simulink model "CubeX_Fast_MPC_2D"  (R2016b)
settings: Solver=FixedStepDiscrete  StartTime=0.0  StopTime=inf  FixedStep=Ts.base  RelTol=1e-3
PreLoadFcn:
  | waijung.modelPreload; % Required for working with Waijung Blockset. Do not remove.
InitFcn:
  | cubeparameters
undefined symbols (not defined in the file or in its folder): CPHA_1Edge, CPOL_Low, deg_, Duplex, FirstBit_MSB, Full, g, imu, Link, LQFP100, ST, STM32F407VG, STM32F4DISCOVERY, Ts
libraries: simulink x47, stm32f4_i2c_lib x12, stm32f4_io_lib x5, stm32f4_spi_lib x4, cube_lib x3, BC_USB x2, stm32f4_adc_lib x1, stm32f4_device_config_lib x1
(part 1 of 3)
CloseFcn:
  | waijung.modelClose; % Required for working with Waijung Blockset. Do not remove.
settings Model: Creator=Hi  LastModifiedBy=Wall
settings DataIOCC: LimitDataPoints=on  SaveFormat=Array
settings OptimizationCC: LifeSpan=1
settings DebuggingCC: AllowSymbolicDim=off  SFUnexpectedBacktrackingDiag=warning  SFNoUnconditionalDefaultTransitionDiag=warning  SFExecutionAtInitializationDiag=none
settings HardwareCC: ProdBitPerPointer=32  ProdBitPerSizeT=32  ProdBitPerPtrDiffT=32  ProdLargestAtomicFloat=None  ProdIntDivRoundTo=Undefined  ProdWordSize=32  ProdHWDeviceType=ARM Compatible->Cortex - M4  TargetEndianess=LittleEndian  TargetHWDeviceType=ARM Compatible->Cortex - M4
settings ModelReferenceCC: PropagateSignalLabelsOutOfModel=off
settings RTWCC: SystemTargetFile=stm32f4.tlc  GenerateMakefile=off  TemplateMakefile=ert_default_tmf  Description=STM32F4 Target
settings CodeAppCC: ForceParamTrailComments=on  IgnoreCustomStorageClasses=off  OperatorAnnotations=on  SimulinkDataObjDesc=on  InsertBlockDesc=on  MATLABSourceComments=on
settings STFCustomTargetCC: ModelReferenceCompliant=off  CombineOutputUpdateFcns=on  ERTCustomFileBanners=on  SupportContinuousTime=off  SupportNonInlinedSFcns=off  RemoveResetFunc=on  MATLABClassNameForMDSCustomization=Simulink.SoftwareTarget.ERTCustomization  GRTInterface=off  SystemTargetFile=stm32f4.tlc
settings ERTTargetCC: ModelReferenceCompliant=off  ParMdlRefBuildCompliant=off  CompOptLevelCompliant=off  ConcurrentExecutionCompliant=off  ERTFirstTimeCompliant=off  ModelStepFunctionPrototypeControlCompliant=off  CPPClassGenCompliant=off  UseToolchainInfoCompliant=off  ERTSrcFileBannerTemplate=stm32f4_code_template.cgt  ERTHdrFileBannerTemplate=stm32f4_code_template.cgt  ERTDataSrcFileTemplate=stm32f4_code_template.cgt  ERTDataHdrFileTemplate=stm32f4_code_template.cgt  ERTCustomFileTemplate=stm32f4_file_process.tlc  ConvertIfToSwitch=off  SuppressUnreachableDefaultCases=off
settings ConfigComp: CovMetricSettings=dw  CovHtmlReporting=on  CovSaveCumulativeToWorkspaceVar=on  CovSaveSingleToWorkspaceVar=on  CovExternalEMLEnable=off

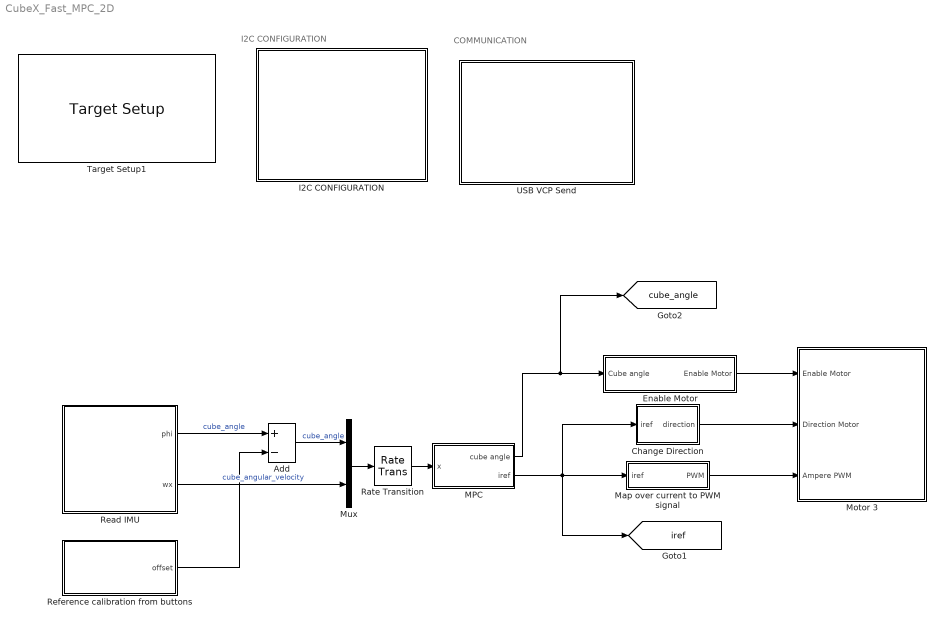
== system CubeX_Fast_MPC_2D ==
  note: COMMUNICATION
  note: I2C CONFIGURATION
  Add : Sum  Inputs=+-
  Change Direction : Subsystem
  Enable Motor : Subsystem  SystemSampleTime=Ts.controller
  I2C CONFIGURATION : Subsystem
  MPC : Subsystem  SystemSampleTime=Ts.controller
      settings: MinAlgLoopOccurrences=on
  Map over current to PWM signal : Subsystem
  Motor 3 : Subsystem
  Mux : Mux  Inputs=2
  Rate Transition : RateTransition  OutPortSampleTime=Ts.controller
  Read IMU : Subsystem
  Reference calibration from buttons : Subsystem
  Target Setup1 : stm32f4_device_config_lib/Target Setup  Priority=100  compiler=GNU ARM  previous_compiler=GNU ARM  mcu=STM32F407VG (LQFP100); STM32F4DISCOVERY  mcustr=STM32F407VG  clockconfig=STM32F4DISCOVERY Default (HSEOSC-8MHz/HCLK-168MHz)  system_stm32f4xx_c_path=C:\waijung15_04a\targets\stm32f4_target\stm32f4\utils\STM32F4xx_AN3988_V1.0.1\stm32f4_default\hseosc8mhz  showmemoryconfiguration=off  stacksize=0x400  heapsize=0x200  enableautocompiledownload=on  fullchiperase=off  programmerinterface=ST-Link  editctrlstr=on  compilercontrolstr=$(patsubst %, -I%, .) -mcpu=cortex-m4 -mthumb -mthumb-interwork -mfloat-abi=hard -mfpu=fpv4-sp-d16 -ffast-math -Wall -Wextra -Ofast  assemblercontrolstr=$(patsubst %, -I%, .) -mcpu=cortex-m4 -mthumb -mthumb-interwork -mfloat-abi=hard -mfpu=fpv4-sp-d16 -ffast-math -Wall -Wextra -Ofast -Wa,-amhls=$(<:.s=.lst) -D__STACK_SIZE=$(STACK_SIZE) -D__HEAP_SIZE=$(HEAP_SIZE)  linkercontrolstr=-T$(LD_SCRIPT) -g -Wl,-Map=$(MAP),--cref,--no-warn-mismatch -mcpu=cortex-m4 -mthumb -mthumb-interwork -mfloat-abi=hard -mfpu=fpv4-sp-d16  runafterdownload=on  execprofile=None  profileruart=1  profilerbaud=115200  profilertxpin=Not used  profilerinitstr=0.002,168000000,336000,115200,0  manualsetsampletime=on  sampletime=0.002  blockid=TargetSetup1  systickreloadvalue=336000  hseval=8000000  lastprofileruart=1  hclk=168000000  flashorigin=0x8000000  flashlength=1M  ramorigin=0x20000000  ramlength=112k  useextram=off
  USB VCP Send : Subsystem
  tag scope: cube_angle=global, iref=global
  wires:
  Read IMU/2(wx) -> Mux/2  "cube_angular_velocity"
  Reference calibration from buttons/1(offset) -> Add/2
  Add/1 -> Mux/1  "cube_angle"
  Read IMU/1(phi) -> Add/1  "cube_angle"
  MPC/2(iref) -> [iref], Change Direction/1(iref), Map over current to PWM signal/1(iref)
  Map over current to PWM signal/1(PWM) -> Motor 3/3(Ampere PWM)
  Change Direction/1(direction) -> Motor 3/2("Direction Motor ")
  Enable Motor/1(Enable Motor) -> Motor 3/1(Enable Motor)
  Mux/1 -> Rate Transition/1
  Rate Transition/1 -> MPC/1(x)
  MPC/1(cube angle) -> [cube_angle], Enable Motor/1(Cube angle)

== system CubeX_Fast_MPC_2D/Change Direction ==
  iref : Inport
  Compare To Zero : simulink/Logic and Bit Operations/Compare To Zero  relop=<=  OutDataTypeStr=boolean
  Logical Operator : Logic  Operator=NOT  AllPortsSameDT=off  OutDataTypeStr=boolean
  direction : Outport
  wires:
  Compare To Zero/1 -> Logical Operator/1
  iref/1 -> Compare To Zero/1
  Logical Operator/1 -> direction/1

== system CubeX_Fast_MPC_2D/Enable Motor ==
  note: When the angle is abs of 6 degrees, Motor is enabled
  Cube angle : Inport
  Abs1 : Abs
  Compare To Constant : simulink/Logic and Bit Operations/Compare To Constant  relop=<=  const=deg2rad(3)  OutDataTypeStr=boolean
  Enable Motor : Outport
  wires:
  Abs1/1 -> Compare To Constant/1
  Cube angle/1 -> Abs1/1
  Compare To Constant/1 -> Enable Motor/1

== system CubeX_Fast_MPC_2D/I2C CONFIGURATION ==
  I2C Master Setup1 : S-Function  FunctionName=stm32f4_i2c  Parameters=configuration,module,transfer,clkspeed,timeout,sdapin,sclpin,writecount,readcount,inputtypearray,outputtypearray,confstr,sampletime,sampletimestr,blockid  SFunctionDeploymentMode=off  EnableBusSupport=off  mask(stm32f4_i2c){configuration=Setup, module=3, lastmodule=3, transfer=Blocking, dutycycle=TLow/THigh = 2, clkspeed=400, timeout=25, writecount=0, readcount=0, sdapin=C9, sclpin=A8, waitwritetime=0, inputtypearray=[0], outputtypearray=[0], confstr=["C","9","A","8","1","3","4","2","I2C_DutyCycle_2","0","off"], sampletime=-1, sampletimestr=0.002, blockid=I2CCONFIGURATIONI2CMasterSetup1}
      mask prompts: module "I2C Module"; lastmodule "Last module"; transfer "Transfer mode"; dutycycle "Duty cycle in fast mode"; clkspeed "Clock speed (kHz)"; timeout "Timeout (ms)"; writecount "Bytes write count"; readcount "Bytes read count"; sdapin "SDA pin"; sclpin "SCL pin"; waitwritetime "Wait write time (ms), default is 0"; inputtypearray "Input type array"; outputtypearray "Output type array"; confstr "Configuration string"; sampletime "Sample time (sec)"; sampletimestr "Compiled sample time (sec) in string"
      mask init:
      | stm32f4_i2c_callback('init');
      mask Help: web(fullfile(waijungdocroot,'stm32f4_i2c_setup.htm'), '-browser')
      mask TypeOptions configuration: Setup | Transaction
      mask Callback configuration: stm32f4_i2c_callback('configuration');
      mask TypeOptions module: 1 | 2 | 3
      mask Callback module: stm32f4_i2c_callback('module');
      mask TypeOptions transfer: Blocking | Non-blocking
      mask TypeOptions dutycycle: TLow/THigh = 16/9 | TLow/THigh = 2
      mask Callback dutycycle: stm32f4_i2c_callback('dutycycle');
      mask Callback writecount: stm32f4_i2c_callback('writecount');
      mask Callback readcount: stm32f4_i2c_callback('readcount');
      mask TypeOptions sdapin: - | C9
      mask Callback sdapin: stm32f4_i2c_callback('sdapin');
      mask TypeOptions sclpin: - | A8
      mask Callback sclpin: stm32f4_i2c_callback('sclpin');
      mask Callback confstr: stm32f4_i2c_callback('confstr');
      mask Callback sampletime: stm32f4_i2c_callback('sampletime');
      mask Callback sampletimestr: stm32f4_i2c_callback('sampletimestr');
      mask Callback blockid: stm32f4_i2c_callback('blockid');
      mask Display: text(0.5, 0.5, 'Module: I2C3\nClock: 400kHz\nSDA/SCL Pin: C9/A8','ver','middle','hor','center');
  I2C Master Setup2 : S-Function  FunctionName=stm32f4_i2c  Parameters=configuration,module,transfer,clkspeed,timeout,sdapin,sclpin,writecount,readcount,inputtypearray,outputtypearray,confstr,sampletime,sampletimestr,blockid  SFunctionDeploymentMode=off  EnableBusSupport=off  mask(stm32f4_i2c){configuration=Setup, module=1, lastmodule=1, transfer=Blocking, dutycycle=TLow/THigh = 2, clkspeed=400, timeout=25, writecount=0, readcount=0, sdapin=B9, sclpin=B6, waitwritetime=0, inputtypearray=[0], outputtypearray=[0], confstr=["B","9","B","6","1","1","6","0","I2C_DutyCycle_2","0","off"], sampletime=-1, sampletimestr=0.002, blockid=I2CCONFIGURATIONI2CMasterSetup2}
      mask prompts: module "I2C Module"; lastmodule "Last module"; transfer "Transfer mode"; dutycycle "Duty cycle in fast mode"; clkspeed "Clock speed (kHz)"; timeout "Timeout (ms)"; writecount "Bytes write count"; readcount "Bytes read count"; sdapin "SDA pin"; sclpin "SCL pin"; waitwritetime "Wait write time (ms), default is 0"; inputtypearray "Input type array"; outputtypearray "Output type array"; confstr "Configuration string"; sampletime "Sample time (sec)"; sampletimestr "Compiled sample time (sec) in string"
      mask init:
      | stm32f4_i2c_callback('init');
      mask Help: web(fullfile(waijungdocroot,'stm32f4_i2c_setup.htm'), '-browser')
      mask TypeOptions configuration: Setup | Transaction
      mask Callback configuration: stm32f4_i2c_callback('configuration');
      mask TypeOptions module: 1 | 2 | 3
      mask Callback module: stm32f4_i2c_callback('module');
      mask TypeOptions transfer: Blocking | Non-blocking
      mask TypeOptions dutycycle: TLow/THigh = 16/9 | TLow/THigh = 2
      mask Callback dutycycle: stm32f4_i2c_callback('dutycycle');
      mask Callback writecount: stm32f4_i2c_callback('writecount');
      mask Callback readcount: stm32f4_i2c_callback('readcount');
      mask TypeOptions sdapin: - | B7 | B9
      mask Callback sdapin: stm32f4_i2c_callback('sdapin');
      mask TypeOptions sclpin: - | B6 | B8
      mask Callback sclpin: stm32f4_i2c_callback('sclpin');
      mask Callback confstr: stm32f4_i2c_callback('confstr');
      mask Callback sampletime: stm32f4_i2c_callback('sampletime');
      mask Callback sampletimestr: stm32f4_i2c_callback('sampletimestr');
      mask Callback blockid: stm32f4_i2c_callback('blockid');
      mask Display: text(0.5, 0.5, 'Module: I2C1\nClock: 400kHz\nSDA/SCL Pin: B9/B6','ver','middle','hor','center');

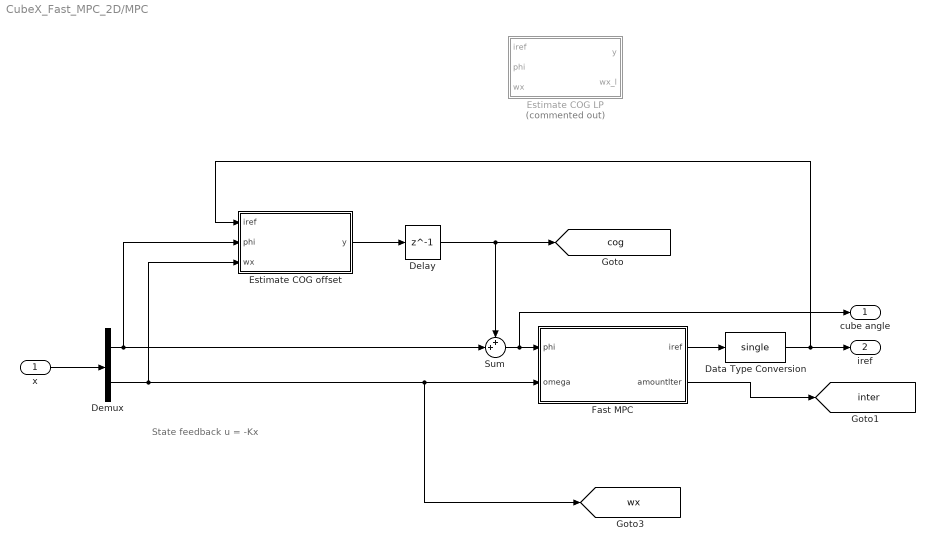
== system CubeX_Fast_MPC_2D/MPC ==
  note: State feedback
      |
      | u = -Kx
  x : Inport
  Data Type Conversion : DataTypeConversion  OutDataTypeStr=single
  Delay : Delay  DelayLength=1
  Demux : Demux  Outputs=2
  Estimate COG LP : MATLAB Function  Commented=on  TreatAsAtomicUnit=on
  Estimate COG offset : MATLAB Function  TreatAsAtomicUnit=on
  Fast MPC : MATLAB Function  TreatAsAtomicUnit=on
  Sum : Sum  Inputs=++|
  cube angle : Outport
  iref : Outport  Port=2
  tag scope: cog=global, inter=global, wx=global
  wires:
  x/1 -> Demux/1
  Demux/2 -> Estimate COG offset/3(wx), [wx], Fast MPC/2(omega)
  Estimate COG offset/1(y) -> Delay/1
  Demux/1 -> Estimate COG offset/2(phi), Sum/2
  Delay/1 -> Sum/1, [cog]
  Sum/1 -> cube angle/1, Fast MPC/1(phi)
  Fast MPC/1(iref) -> Data Type Conversion/1
  Data Type Conversion/1 -> Estimate COG offset/1(iref), iref/1
  Fast MPC/2(amountIter) -> [inter]

== system CubeX_Fast_MPC_2D/Map over current to PWM signal ==
  note: Map over current to duty
      | current limit: 0-4A
      | duty limit: 10-90%
      |
      | (90-10) / (4-0) = 20 -> k
      | 10 -> m
  iref : Inport
  Abs : Abs
  Add : Sum
  Saturation on duty : Saturate  UpperLimit=90  LowerLimit=10  OutDataTypeStr=single
  k : Gain  Gain=20
  m : Constant  Value=10  OutDataTypeStr=single  SampleTime=Ts.controller
  PWM : Outport
  wires:
  Add/1 -> Saturation on duty/1
  Saturation on duty/1 -> PWM/1
  iref/1 -> Abs/1
  Abs/1 -> k/1
  k/1 -> Add/1
  m/1 -> Add/2

== system CubeX_Fast_MPC_2D/Motor 3 ==
  Enable Motor : Inport
  "Direction Motor " : Inport  Port=2
  Ampere PWM : Inport  Port=3
  Direction Motor 3 (green) : stm32f4_io_lib/Digital Output  use_bitband=on  port=D  speed=100  porttype=Push Pull  porttypestr=PP  use_pin0=off  use_pin1=off  use_pin2=off  use_pin3=off  use_pin4=off  use_pin5=off  use_pin6=off  use_pin7=off  use_pin8=off  use_pin9=off  use_pin10=off  use_pin11=on  use_pin12=off  use_pin13=off  use_pin14=off  use_pin15=off  pinstr=GPIO_Pin_11  usedpinarray="[0  0  0  0  0  0  0  0  0  0  0  1  0  0  0  0]"  bitbandingstr="#define Motor3DirectionMotor3green_D11 Peripheral_BB(GPIOD->ODR, 11)  /* Output pin */"  sampletime=-1  sampletimestr=0.056  blockid=Motor3DirectionMotor3green  enablecustomportlabel=off  globalinit=off  cinputportlabel=In1, In2  coutputportlabel=0
  Enable Motor 3(yellow) : stm32f4_io_lib/Digital Output  use_bitband=on  port=D  speed=100  porttype=Push Pull  porttypestr=PP  use_pin0=off  use_pin1=off  use_pin2=off  use_pin3=off  use_pin4=off  use_pin5=off  use_pin6=off  use_pin7=off  use_pin8=off  use_pin9=on  use_pin10=off  use_pin11=off  use_pin12=off  use_pin13=off  use_pin14=off  use_pin15=off  pinstr=GPIO_Pin_9  usedpinarray="[0  0  0  0  0  0  0  0  0  1  0  0  0  0  0  0]"  bitbandingstr="#define Motor3EnableMotor3yellow_D9 Peripheral_BB(GPIOD->ODR, 9)  /* Output pin */"  sampletime=-1  sampletimestr=0.056  blockid=Motor3EnableMotor3yellow  enablecustomportlabel=off  globalinit=off  cinputportlabel=In1, In2  coutputportlabel=0
  PWM Ampere motor 1 : S-Function  Commented=on  FunctionName=stm32f4_basicpwm_fixed  Parameters=timer,pwmperiod,uc3m_pwmperiod,ch1pin,ch2pin,ch3pin,ch4pin,sampletime,sampletimestr,blockid,apb,portstr,pinstr,pinmat,timarr,timprescale,chmat,polaritystr  SFunctionDeploymentMode=off  EnableBusSupport=off  mask(stm32f4_basicpwm_fixed){timer=5, pwmperiod=0.02, uc3m_pwmperiod=0.0002, polarity=Active High, polaritystr=TIM_OCPolarity_High, ch1pin=Not available - Do not use, ch2pin=Not available - Do not use, ch3pin=Not available - Do not use, ch4pin=A3, sampletime=0.002, sampletimestr=0.002, blockid=motor3PWMAmperemotor3, portpinstr=,,,A3, enablecustomportlabel=off, cinputportlabel=In1, In2, In3, In4, coutputportlabel=0, callbackgensrccode=off, apb=1, portstr=["A"], pinstr=["GPIO_Pin_3"], pinmat=[1 3], timarr=59999, timprescale=55, chmat=[4]}
      mask prompts: pwmperiod "PWM Period (seconds)"; uc3m_pwmperiod "PWM Signal Period (seconds)"; ch1pin "Channel 1"; ch2pin "Channel 2"; ch3pin "Channel 3"; ch4pin "Channel 4"; sampletime "Sample time (sec)"; sampletimestr "Compiled sample time (sec) in string"; portpinstr "Port pin string"; enablecustomportlabel "Enable custom port labels"; cinputportlabel "Custom input port labels (Ex. In1, In2, In3)"; coutputportlabel "Custom output port labels (Ex. Out1, Out2, Out3)"; callbackgensrccode "Gen source code from callback"; portstr "Port string"; pinstr "Pin string"; pinmat "Pin matrix"; timarr "Timer ARR"; timprescale "Timer PRESCALE"; chmat "Channel order"
      mask help:
      | This block implements basic Edge-aligned Pulse Width Modulation (PWM) generation.
      | All timers are 16-bit. The PWM period is fixed (per timer).
      |
      | This block was fixed by Sr Antonio
      mask init:
      | stm32f4_basicpwm_callback_fixed('init');
      mask Help: web(fullfile(waijungdocroot,'stm32f4_basicpwm.htm'),'-browser')
      mask TypeOptions timer: 1 | 2 | 3 | 4 | 5 | 8 | 9 | 10 | 11 | 12 | 13 | 14
      mask Callback timer: stm32f4_basicpwm_callback_fixed('timer');
      mask Callback pwmperiod: stm32f4_basicpwm_callback_fixed('pwmperiod');
      mask Callback uc3m_pwmperiod: stm32f4_basicpwm_callback_fixed('uc3m_pwmperiod');
      mask TypeOptions polarity: Active High | Active Low
      mask Callback polarity: stm32f4_basicpwm_callback_fixed('polarity');
      mask TypeOptions ch1pin: Not available - Do not use | A0 | A5
      mask Callback ch1pin: stm32f4_basicpwm_callback_fixed('ch1pin');
      mask TypeOptions ch2pin: Not available - Do not use | A1 | B3
      mask Callback ch2pin: stm32f4_basicpwm_callback_fixed('ch2pin');
      mask TypeOptions ch3pin: Not available - Do not use | A2 | B10
      mask Callback ch3pin: stm32f4_basicpwm_callback_fixed('ch3pin');
      mask TypeOptions ch4pin: Not available - Do not use | A3 | B11
      mask Callback ch4pin: stm32f4_basicpwm_callback_fixed('ch4pin');
      mask Callback sampletime: stm32f4_basicpwm_callback_fixed('sampletime');
      mask Callback sampletimestr: stm32f4_basicpwm_callback_fixed('sampletimestr');
      mask Callback blockid: stm32f4_basicpwm_callback_fixed('blockid');
      mask Callback enablecustomportlabel: stm32f4_basicpwm_callback_fixed('enablecustomportlabel')
      mask Display: text(0.95, 0.5, 'UC3M FIXED\nTimer: 5\nPolarity: Active High\nPeriod (sec): 0.0002\nTs (sec): 0.002','ver','middle','hor','right');port_label('input', 1,'CH4 (A3)')
  PWM Ampere motor 3 : S-Function  FunctionName=stm32f4_basicpwm_fixed  Parameters=timer,pwmperiod,uc3m_pwmperiod,ch1pin,ch2pin,ch3pin,ch4pin,sampletime,sampletimestr,blockid,apb,portstr,pinstr,pinmat,timarr,timprescale,chmat,polaritystr  SFunctionDeploymentMode=off  EnableBusSupport=off  mask(stm32f4_basicpwm_fixed){timer=2, pwmperiod=0.02, uc3m_pwmperiod=0.0002, polarity=Active High, polaritystr=TIM_OCPolarity_High, ch1pin=Not available - Do not use, ch2pin=Not available - Do not use, ch3pin=Not available - Do not use, ch4pin=A3, sampletime=-1, sampletimestr=0.056, blockid=Motor3PWMAmperemotor3, portpinstr=,,,A3, enablecustomportlabel=off, cinputportlabel=In1, In2, In3, In4, coutputportlabel=0, callbackgensrccode=off, apb=1, portstr=["A"], pinstr=["GPIO_Pin_3"], pinmat=[1 3], timarr=59999, timprescale=55, chmat=[4]}
      mask prompts: pwmperiod "PWM Period (seconds)"; uc3m_pwmperiod "PWM Signal Period (seconds)"; ch1pin "Channel 1"; ch2pin "Channel 2"; ch3pin "Channel 3"; ch4pin "Channel 4"; sampletime "Sample time (sec)"; sampletimestr "Compiled sample time (sec) in string"; portpinstr "Port pin string"; enablecustomportlabel "Enable custom port labels"; cinputportlabel "Custom input port labels (Ex. In1, In2, In3)"; coutputportlabel "Custom output port labels (Ex. Out1, Out2, Out3)"; callbackgensrccode "Gen source code from callback"; portstr "Port string"; pinstr "Pin string"; pinmat "Pin matrix"; timarr "Timer ARR"; timprescale "Timer PRESCALE"; chmat "Channel order"
      mask help:
      | This block implements basic Edge-aligned Pulse Width Modulation (PWM) generation.
      | All timers are 16-bit. The PWM period is fixed (per timer).
      |
      | This block was fixed by Sr Antonio
      mask init:
      | stm32f4_basicpwm_callback_fixed('init');
      mask Help: web(fullfile(waijungdocroot,'stm32f4_basicpwm.htm'),'-browser')
      mask TypeOptions timer: 1 | 2 | 3 | 4 | 5 | 8 | 9 | 10 | 11 | 12 | 13 | 14
      mask Callback timer: stm32f4_basicpwm_callback_fixed('timer');
      mask Callback pwmperiod: stm32f4_basicpwm_callback_fixed('pwmperiod');
      mask Callback uc3m_pwmperiod: stm32f4_basicpwm_callback_fixed('uc3m_pwmperiod');
      mask TypeOptions polarity: Active High | Active Low
      mask Callback polarity: stm32f4_basicpwm_callback_fixed('polarity');
      mask TypeOptions ch1pin: Not available - Do not use | A0 | A5
      mask Callback ch1pin: stm32f4_basicpwm_callback_fixed('ch1pin');
      mask TypeOptions ch2pin: Not available - Do not use | A1 | B3
      mask Callback ch2pin: stm32f4_basicpwm_callback_fixed('ch2pin');
      mask TypeOptions ch3pin: Not available - Do not use | A2 | B10
      mask Callback ch3pin: stm32f4_basicpwm_callback_fixed('ch3pin');
      mask TypeOptions ch4pin: Not available - Do not use | A3 | B11
      mask Callback ch4pin: stm32f4_basicpwm_callback_fixed('ch4pin');
      mask Callback sampletime: stm32f4_basicpwm_callback_fixed('sampletime');
      mask Callback sampletimestr: stm32f4_basicpwm_callback_fixed('sampletimestr');
      mask Callback blockid: stm32f4_basicpwm_callback_fixed('blockid');
      mask Callback enablecustomportlabel: stm32f4_basicpwm_callback_fixed('enablecustomportlabel')
      mask Display: text(0.95, 0.5, 'UC3M FIXED\nTimer: 2\nPolarity: Active High\nPeriod (sec): 0.0002\nTs (sec): -1','ver','middle','hor','right');port_label('input', 1,'CH4 (A3)')
  "Velocty wheel 3, analog in (Grey), PC1" : stm32f4_adc_lib/Regular ADC  Commented=on  adcmodule=3  outputdatatype=Single  prescaler=2  prescalerstr=ADC_Prescaler_Div2  chsamplingtime=Auto  chsamplingtimestr=ADC_SampleTime_480Cycles  read_an0=off  read_an1=off  read_an2=off  read_an3=off  read_an4=off  read_an5=off  read_an6=off  read_an7=off  read_an8=off  read_an9=off  read_an10=on  read_an11=off  read_an12=off  read_an13=off  read_an14=off  read_an15=off  read_an16=off  read_an17=off  read_an18=off  pinstr=GPIO_Pin_10  usedpinarray="[0  0  0  0  0  0  0  0  0  0  1  0  0  0  0  0  0  0  0]"  usedportidarray=[2]  usedpinidarray=[0]  usedpinidcount=1  sampletime=0.002  blockid=Motor3Veloctywheel3analoginGreyPC1  enablecustomportlabel=off  cinputportlabel=0  coutputportlabel=Out1, Out2
  wires:
  Ampere PWM/1 -> PWM Ampere motor 3/1
  "Direction Motor "/1 -> Direction Motor 3 (green)/1
  Enable Motor/1 -> Enable Motor 3(yellow)/1

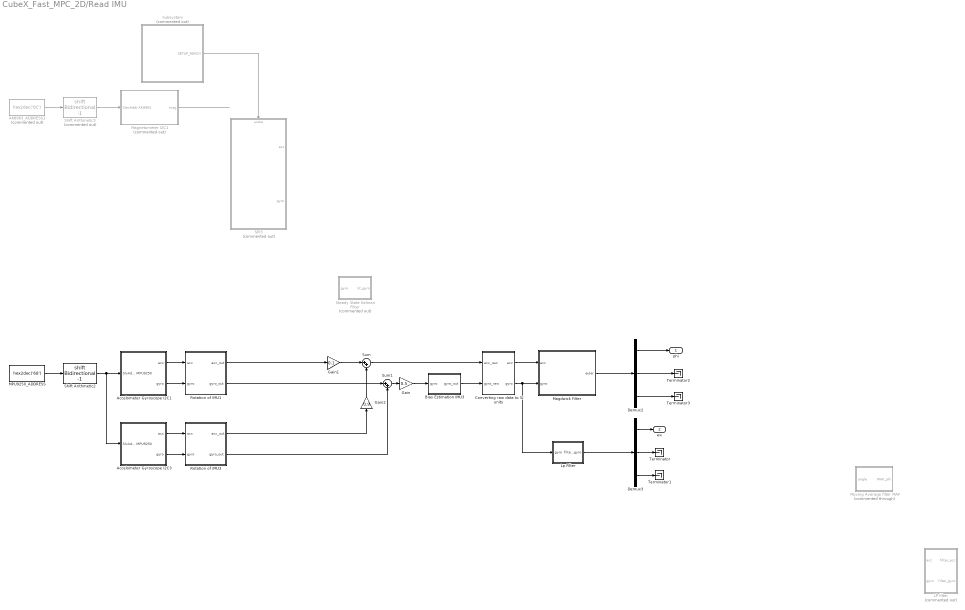
== system CubeX_Fast_MPC_2D/Read IMU ==
  " AK8963_ADDRESS1" : Constant  Commented=on  Value=hex2dec('0C')  OutDataTypeStr=uint8  SampleTime=0.002
  " MPU9250_ADDRESS" : Constant  Value=hex2dec('68')  OutDataTypeStr=uint8  SampleTime=Ts.IMU
  Accelometer Gyroscope I2C1 : Subsystem
  Accelometer Gyroscope I2C3 : Subsystem
  Bias Estimation IMU3 : MATLAB Function  TreatAsAtomicUnit=on
  Converting raw data to SI units : Subsystem
  Demux2 : Demux  Outputs=3
  Demux3 : Demux  Outputs=3
  Gain : Gain  Gain=0.5
  Gain1 : Gain  Gain=0.1
  Gain2 : Gain  Gain=0.9
  LP filter : MATLAB Function  Commented=on  TreatAsAtomicUnit=on
  Lp Filter : MATLAB Function  TreatAsAtomicUnit=on
  Magdwick Filter : MATLAB Function  TreatAsAtomicUnit=on
  Magnetometer I2C1 : Subsystem  Commented=on
  Moving Average filter MAF : MATLAB Function  Commented=through  TreatAsAtomicUnit=on
  Rotation of IMU1 : MATLAB Function  TreatAsAtomicUnit=on
  Rotation of IMU3 : MATLAB Function  TreatAsAtomicUnit=on
  SPI3 : Subsystem  Commented=on
  Shift Arithmetic2 : ArithShift  BitShiftNumber=-1
  Shift Arithmetic3 : ArithShift  Commented=on  BitShiftNumber=-1
  Steady State Kalman Filter : MATLAB Function  Commented=on  TreatAsAtomicUnit=on
  Subsystem : Subsystem  Commented=on
  Sum : Sum  Inputs=|++
  Sum1 : Sum  Inputs=|++
  Terminator{,1..3} (4 alike) : Terminator
  phi : Outport
  wx : Outport  Port=2
  wires:
  Demux3/2 -> Terminator/1
  Demux2/2 -> Terminator2/1
  Demux2/3 -> Terminator3/1
  Demux3/3 -> Terminator1/1
  Demux2/1 -> phi/1
  Converting raw data to SI units/1(acc) -> Magdwick Filter/1(acc)
  Demux3/1 -> wx/1
  Lp Filter/1(filter_gyro) -> Demux3/1
  Magdwick Filter/1(euler) -> Demux2/1
  Converting raw data to SI units/2(gyro) -> Magdwick Filter/2(gyro), Lp Filter/1(gyro)
  Accelometer Gyroscope I2C1/2(gyro) -> Rotation of IMU1/2(gyro)
  Subsystem/1(SETUP_READY) -> SPI3/Enable
  Shift Arithmetic2/1 -> Accelometer Gyroscope I2C3/1(SlvAddr MPU9250), Accelometer Gyroscope I2C1/1(SlvAddr MPU9250)
  Accelometer Gyroscope I2C1/1(acc) -> Rotation of IMU1/1(acc)
  " MPU9250_ADDRESS"/1 -> Shift Arithmetic2/1
  Shift Arithmetic3/1 -> Magnetometer I2C1/1(SlavAddr AK8963)
  " AK8963_ADDRESS1"/1 -> Shift Arithmetic3/1
  Magnetometer I2C1/1(mag) -> ?
  Accelometer Gyroscope I2C3/1(acc) -> Rotation of IMU3/1(acc)
  Accelometer Gyroscope I2C3/2(gyro) -> Rotation of IMU3/2(gyro)
  Rotation of IMU1/1(acc_out) -> Gain1/1
  Rotation of IMU3/1(acc_out) -> Gain2/1
  Sum1/1 -> Gain/1
  Gain/1 -> Bias Estimation IMU3/1(gyro)
  Sum/1 -> Converting raw data to SI units/1(acc_raw)
  Rotation of IMU3/2(gyro_out) -> Sum1/2
  Rotation of IMU1/2(gyro_out) -> Sum1/1
  Gain2/1 -> Sum/2
  Gain1/1 -> Sum/1
  Bias Estimation IMU3/1(gyro_out) -> Converting raw data to SI units/2(gyro_raw)

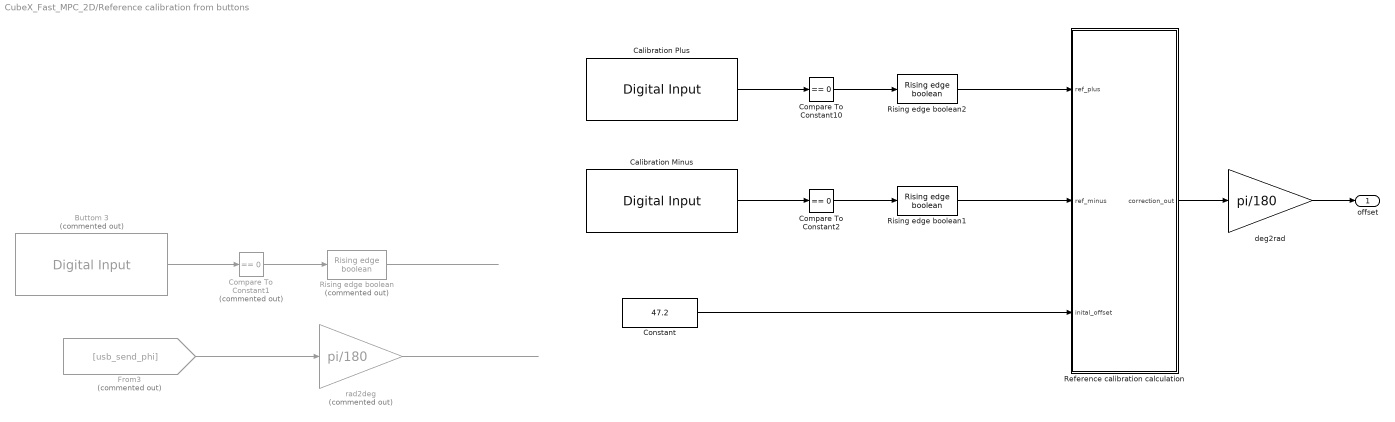
== system CubeX_Fast_MPC_2D/Reference calibration from buttons ==
  Buttom 3 : stm32f4_io_lib/Digital Input  Commented=on  port=E  speed=100  porttype=Pull Up  porttypestr=UP  use_pin0=off  use_pin1=off  use_pin2=off  use_pin3=off  use_pin4=off  use_pin5=off  use_pin6=off  use_pin7=off  use_pin8=off  use_pin9=off  use_pin10=on  use_pin11=off  use_pin12=off  use_pin13=off  use_pin14=off  use_pin15=off  pinstr=GPIO_Pin_10  usedpinarray="[0  0  0  0  0  0  0  0  0  0  1  0  0  0  0  0]"  bitbandingstr="#define ReferencecalibrationfrombuttonsButtom3_E10 Peripheral_BB(GPIOE->IDR, 10)  /* Output pin */"  sampletime=Ts.IMU  sampletimestr=-1  blockid=ReferencecalibrationfrombuttonsButtom3  enablecustomportlabel=off  glabalinit=off  cinputportlabel=In1, In2  coutputportlabel=Out1, Out2
  Calibration Minus : stm32f4_io_lib/Digital Input  port=E  speed=100  porttype=Pull Up  porttypestr=UP  use_pin0=off  use_pin1=off  use_pin2=off  use_pin3=off  use_pin4=off  use_pin5=off  use_pin6=off  use_pin7=off  use_pin8=off  use_pin9=off  use_pin10=off  use_pin11=off  use_pin12=off  use_pin13=off  use_pin14=on  use_pin15=off  pinstr=GPIO_Pin_14  usedpinarray="[0  0  0  0  0  0  0  0  0  0  0  0  0  0  1  0]"  bitbandingstr="#define ReferencecalibrationfrombuttonsCalibrationMinus_E14 Peripheral_BB(GPIOE->IDR, 14)  /* Output pin */"  sampletime=Ts.IMU  sampletimestr=0.008  blockid=ReferencecalibrationfrombuttonsCalibrationMinus  enablecustomportlabel=off  glabalinit=off  cinputportlabel=In1, In2  coutputportlabel=Out1, Out2
  Calibration Plus : stm32f4_io_lib/Digital Input  port=E  speed=100  porttype=Pull Up  porttypestr=UP  use_pin0=off  use_pin1=off  use_pin2=off  use_pin3=off  use_pin4=off  use_pin5=off  use_pin6=off  use_pin7=off  use_pin8=off  use_pin9=off  use_pin10=off  use_pin11=on  use_pin12=off  use_pin13=off  use_pin14=off  use_pin15=off  pinstr=GPIO_Pin_11  usedpinarray="[0  0  0  0  0  0  0  0  0  0  0  1  0  0  0  0]"  bitbandingstr="#define ReferencecalibrationfrombuttonsCalibrationPlus_E11 Peripheral_BB(GPIOE->IDR, 11)  /* Output pin */"  sampletime=Ts.IMU  sampletimestr=0.008  blockid=ReferencecalibrationfrombuttonsCalibrationPlus  enablecustomportlabel=off  glabalinit=off  cinputportlabel=In1, In2  coutputportlabel=Out1, Out2
  Compare To Constant1 : simulink/Logic and Bit Operations/Compare To Constant  Commented=on  relop===  const=0  OutDataTypeStr=boolean  ZeroCross=off
  Compare To Constant10 : simulink/Logic and Bit Operations/Compare To Constant  relop===  const=0  OutDataTypeStr=boolean  ZeroCross=off
  Compare To Constant2 : simulink/Logic and Bit Operations/Compare To Constant  relop===  const=0  OutDataTypeStr=boolean  ZeroCross=off
  Constant : Constant  Value=47.2  OutDataTypeStr=single  SampleTime=Ts.IMU
  From3 : From  Commented=on  GotoTag=usb_send_phi
  Reference calibration calculation : MATLAB Function  TreatAsAtomicUnit=on
  Rising edge boolean : cube_lib/Rising edge boolean  Commented=on
  Rising edge boolean1 : cube_lib/Rising edge boolean
  Rising edge boolean2 : cube_lib/Rising edge boolean
  deg2rad : Gain  Gain=pi/180  ParamDataTypeStr=single
  rad2deg : Gain  Commented=on  Gain=pi/180  ParamDataTypeStr=single
  offset : Outport
  wires:
  Compare To Constant10/1 -> Rising edge boolean2/1
  Reference calibration calculation/1(correction_out) -> deg2rad/1
  Calibration Minus/1 -> Compare To Constant2/1
  Calibration Plus/1 -> Compare To Constant10/1
  Rising edge boolean1/1 -> Reference calibration calculation/2(ref_minus)
  Compare To Constant2/1 -> Rising edge boolean1/1
  Rising edge boolean2/1 -> Reference calibration calculation/1(ref_plus)
  Compare To Constant1/1 -> Rising edge boolean/1
  Buttom 3/1 -> Compare To Constant1/1
  Rising edge boolean/1 -> ?
  Constant/1 -> Reference calibration calculation/3(inital_offset)
  deg2rad/1 -> offset/1
  From3/1 -> rad2deg/1
  rad2deg/1 -> ?

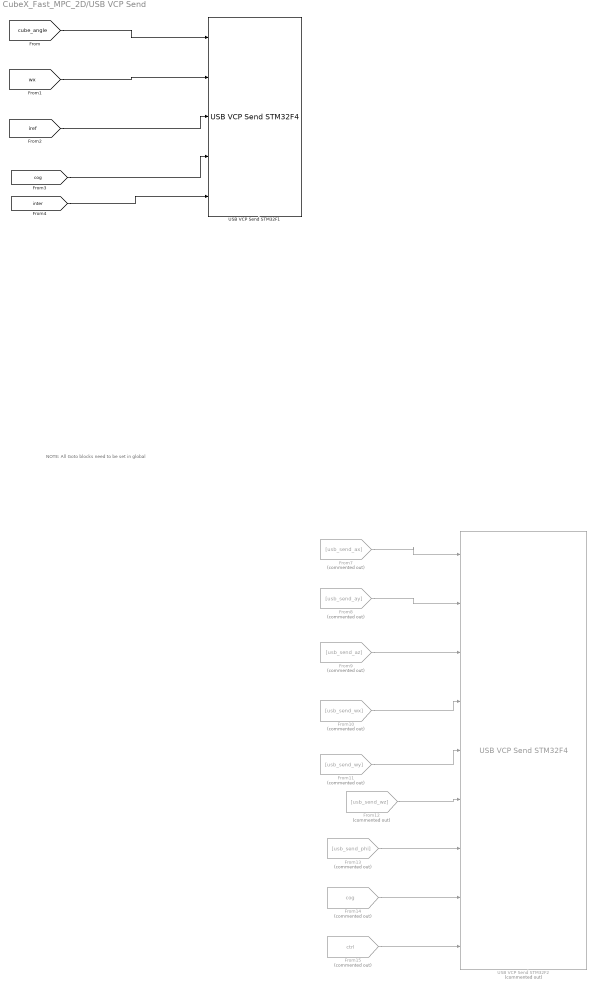
== system CubeX_Fast_MPC_2D/USB VCP Send ==
  note: NOTE: All Goto blocks need to be set in global
  From10 : From  Commented=on  GotoTag=usb_send_wx  TagVisibility=global
  From11 : From  Commented=on  GotoTag=usb_send_wy  TagVisibility=global
  From12 : From  Commented=on  GotoTag=usb_send_wz  TagVisibility=global
  From13 : From  Commented=on  GotoTag=usb_send_phi  TagVisibility=global
  From14 : From  Commented=on  GotoTag=cog  TagVisibility=global
  From15 : From  Commented=on  GotoTag=ctrl
  From7 : From  Commented=on  GotoTag=usb_send_ax  TagVisibility=global
  From8 : From  Commented=on  GotoTag=usb_send_ay  TagVisibility=global
  From9 : From  Commented=on  GotoTag=usb_send_az  TagVisibility=global
  USB VCP Send STM32F1 : BC_USB/USB VCP Send STM32F4  speed="USB 1.1   12Mbit/s"  data_size=2048 Bytes  header_data='0E 0E'  binary_data='single single single single single'  terminator_data='0A 0A'  sampletime=Ts.base
  USB VCP Send STM32F2 : BC_USB/USB VCP Send STM32F4  Commented=on  speed="USB 1.1   12Mbit/s"  data_size=2048 Bytes  header_data='0E 0E'  binary_data='single single single single single single single single single'  terminator_data='0A 0A'  sampletime=Ts.base
  wires:
  [cube_angle] -> USB VCP Send STM32F1/1
  [wx] -> USB VCP Send STM32F1/2
  From7/1 -> USB VCP Send STM32F2/1
  From9/1 -> USB VCP Send STM32F2/3
  From8/1 -> USB VCP Send STM32F2/2
  From10/1 -> USB VCP Send STM32F2/4
  From11/1 -> USB VCP Send STM32F2/5
  From12/1 -> USB VCP Send STM32F2/6
  From13/1 -> USB VCP Send STM32F2/7
  From14/1 -> USB VCP Send STM32F2/8
  From15/1 -> USB VCP Send STM32F2/9
  [iref] -> USB VCP Send STM32F1/3
  [cog] -> USB VCP Send STM32F1/4
  [inter] -> USB VCP Send STM32F1/5

== system CubeX_Fast_MPC_2D/Read IMU/Accelometer Gyroscope I2C1 ==
  SlvAddr MPU9250 : Inport
  MPU9250 Init : Subsystem
  Read Accelometer and Gyroscope Data : Subsystem
  acc : Outport
  gyro : Outport  Port=2
  wires:
  SlvAddr MPU9250/1 -> Read Accelometer and Gyroscope Data/1(SlvAddr), MPU9250 Init/1(SlvAddr)
  Read Accelometer and Gyroscope Data/1(acc) -> acc/1
  Read Accelometer and Gyroscope Data/2(gyro) -> gyro/1
  MPU9250 Init/1(SETUP_READY) -> Read Accelometer and Gyroscope Data/Enable

== system CubeX_Fast_MPC_2D/Read IMU/Accelometer Gyroscope I2C3 ==
  SlvAddr MPU9250 : Inport
  MPU9250 Init : Subsystem
  Read Accelometer and Gyroscope Data : Subsystem
  acc : Outport
  gyro : Outport  Port=2
  wires:
  SlvAddr MPU9250/1 -> Read Accelometer and Gyroscope Data/1(SlvAddr), MPU9250 Init/1(SlvAddr)
  Read Accelometer and Gyroscope Data/1(acc) -> acc/1
  Read Accelometer and Gyroscope Data/2(gyro) -> gyro/1
  MPU9250 Init/1(SETUP_READY) -> Read Accelometer and Gyroscope Data/Enable

== system CubeX_Fast_MPC_2D/Read IMU/Converting raw data to SI units ==
  acc_raw : Inport
  gyro_raw : Inport  Port=2
  Raw sensor value to SI units Accelometer : Gain  Gain=1 / imu.a_scaling * g
  Raw sensor value to SI units Gyroscope : Gain  Gain=1 / imu.w_scaling * deg_
  acc : Outport
  gyro : Outport  Port=2
  wires:
  gyro_raw/1 -> Raw sensor value to SI units Gyroscope/1
  Raw sensor value to SI units Accelometer/1 -> acc/1
  Raw sensor value to SI units Gyroscope/1 -> gyro/1
  acc_raw/1 -> Raw sensor value to SI units Accelometer/1

== system CubeX_Fast_MPC_2D/Read IMU/Magnetometer I2C1 ==
  note: Read magnetometer data for the third party sensor on the MPU9250
  SlavAddr AK8963 : Inport
  "AK8963 Init " : Subsystem
  "Magnetometer Data Ready " : Subsystem
  Read Magnetometer Data : Subsystem
  mag : Outport
  wires:
  "AK8963 Init "/1(READY) -> "Magnetometer Data Ready "/Enable
  Read Magnetometer Data/1(mag) -> mag/1
  SlavAddr AK8963/1 -> "Magnetometer Data Ready "/1(SlvAddr), Read Magnetometer Data/1("SlvAddr "), "AK8963 Init "/1(SlvAddr)
  "Magnetometer Data Ready "/1(READY) -> Read Magnetometer Data/Enable

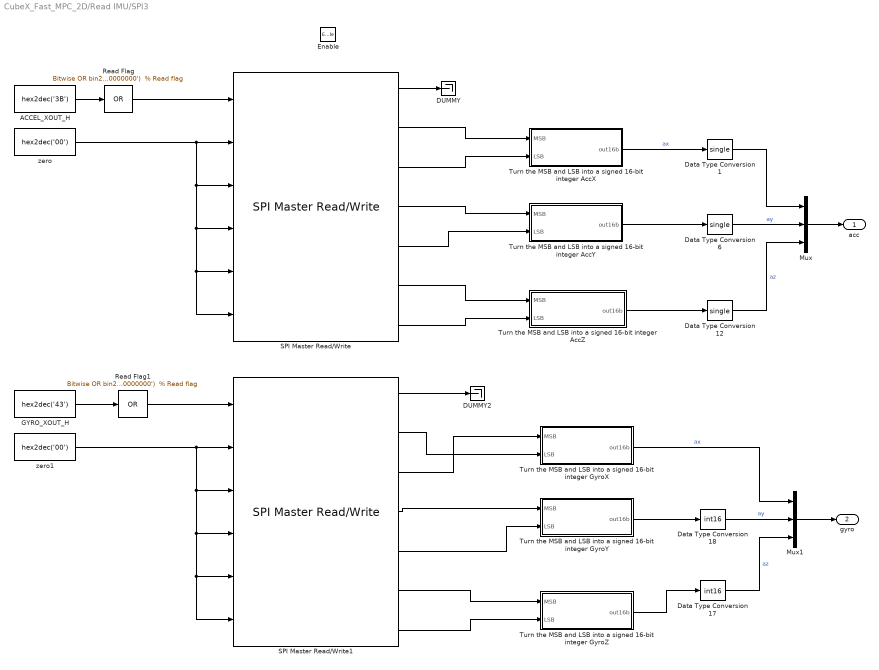
== system CubeX_Fast_MPC_2D/Read IMU/SPI3 ==
  Enable : EnablePort
  ACCEL_XOUT_H : Constant  Value=hex2dec('3B')  OutDataTypeStr=uint8  SampleTime=-1
  DUMMY : Terminator
  DUMMY2 : Terminator
  Data Type Conversion1 : DataTypeConversion  OutDataTypeStr=single
  Data Type Conversion12 : DataTypeConversion  OutDataTypeStr=single
  Data Type Conversion17 : DataTypeConversion  OutDataTypeStr=int16
  Data Type Conversion18 : DataTypeConversion  OutDataTypeStr=int16
  Data Type Conversion6 : DataTypeConversion  OutDataTypeStr=single
  GYRO_XOUT_H : Constant  Value=hex2dec('43')  OutDataTypeStr=uint8  SampleTime=-1
  Mux : Mux  Inputs=3
  Mux1 : Mux  Inputs=3
  Read Flag : simulink/Logic and Bit Operations/Bitwise Operator  logicop=OR  UseBitMask=on  BitMask="bin2dec('10000000')  % Read flag"  BitMaskRealWorld=Real World Value
  Read Flag1 : simulink/Logic and Bit Operations/Bitwise Operator  logicop=OR  UseBitMask=on  BitMask="bin2dec('10000000')  % Read flag"  BitMaskRealWorld=Real World Value
  SPI Master Read/Write : stm32f4_spi_lib/SPI Master Read//Write  configuration=Transaction  module=3  mode=Read/ Write  lastmodule=1  direction=Full-Duplex  dataformat=8bit/ FirstBit_MSB  prescaler=4  cpolcpha=CPOL_Low/ CPHA_1Edge  datacount=6  nssmode=Custom  nsspin=Not used  softnssport=E  softnsspin=0  sckpin=A5  misopin=A6  mosipin=A7  inputtypearray=[6 3 3 3 3 3 3]  outputtypearray=[7 7 3 3 3 3 3 3]  confstr="[\"SPI_Direction_2Lines_FullDuplex\",\"8b\",\"MSB\",\"Low\",\"1Edge\",\"4\",\"Soft\",\"0\",\"x\",\"x\",\"0\",\"x\",\"x\",\"1\",\"A\",\"5\",\"1\",\"A\",\"6\",\"1\",\"A\",\"7\",\"1\",\"0\",\"0\",\"0\",\"0\",\"0\",\"0\",\"0\",\"0\",\"PP\",\"0\",\"UP\"]"  sampletime=0.002  sampletimestr=0.002  blockid=ReadIMUSPI3SPIMasterReadWrite
  SPI Master Read/Write1 : stm32f4_spi_lib/SPI Master Read//Write  configuration=Transaction  module=3  mode=Read/ Write  lastmodule=1  direction=Full-Duplex  dataformat=8bit/ FirstBit_MSB  prescaler=4  cpolcpha=CPOL_Low/ CPHA_1Edge  datacount=6  nssmode=Custom  nsspin=Not used  softnssport=E  softnsspin=0  sckpin=A5  misopin=A6  mosipin=A7  inputtypearray=[6 3 3 3 3 3 3]  outputtypearray=[7 7 3 3 3 3 3 3]  confstr="[\"SPI_Direction_2Lines_FullDuplex\",\"8b\",\"MSB\",\"Low\",\"1Edge\",\"4\",\"Soft\",\"0\",\"x\",\"x\",\"0\",\"x\",\"x\",\"1\",\"A\",\"5\",\"1\",\"A\",\"6\",\"1\",\"A\",\"7\",\"1\",\"0\",\"0\",\"0\",\"0\",\"0\",\"0\",\"0\",\"0\",\"PP\",\"0\",\"UP\"]"  sampletime=0.002  sampletimestr=0.002  blockid=ReadIMUSPI3SPIMasterReadWrite1
  Turn the MSB and LSB into a signed 16-bit integer AccX : Subsystem
  Turn the MSB and LSB into a signed 16-bit integer AccY : Subsystem
  Turn the MSB and LSB into a signed 16-bit integer AccZ : Subsystem
  Turn the MSB and LSB into a signed 16-bit integer GyroX : Subsystem
  Turn the MSB and LSB into a signed 16-bit integer GyroY : Subsystem
  Turn the MSB and LSB into a signed 16-bit integer GyroZ : Subsystem
  zero : Constant  Value=hex2dec('00')  OutDataTypeStr=uint8  SampleTime=-1
  zero1 : Constant  Value=hex2dec('00')  OutDataTypeStr=uint8  SampleTime=-1
  acc : Outport
  gyro : Outport  Port=2
  wires:
  Data Type Conversion6/1 -> Mux/2  "ay"
  Mux1/1 -> gyro/1
  GYRO_XOUT_H/1 -> Read Flag1/1
  SPI Master Read/Write/1 -> DUMMY/1
  SPI Master Read/Write1/1 -> DUMMY2/1
  Mux/1 -> acc/1
  Data Type Conversion18/1 -> Mux1/2  "ay"
  Turn the MSB and LSB into a signed 16-bit integer GyroZ/1(out16b) -> Data Type Conversion17/1
  Turn the MSB and LSB into a signed 16-bit integer AccX/1(out16b) -> Data Type Conversion1/1  "ax"
  Turn the MSB and LSB into a signed 16-bit integer GyroY/1(out16b) -> Data Type Conversion18/1
  Turn the MSB and LSB into a signed 16-bit integer GyroX/1(out16b) -> Mux1/1  "ax"
  Turn the MSB and LSB into a signed 16-bit integer AccY/1(out16b) -> Data Type Conversion6/1
  Turn the MSB and LSB into a signed 16-bit integer AccZ/1(out16b) -> Data Type Conversion12/1
  Data Type Conversion12/1 -> Mux/3  "az"
  Data Type Conversion17/1 -> Mux1/3  "az"
  ACCEL_XOUT_H/1 -> Read Flag/1
  Read Flag/1 -> SPI Master Read/Write/1
  zero/1 -> SPI Master Read/Write/6, SPI Master Read/Write/5, SPI Master Read/Write/4, SPI Master Read/Write/3, SPI Master Read/Write/2
  Read Flag1/1 -> SPI Master Read/Write1/1
  zero1/1 -> SPI Master Read/Write1/6, SPI Master Read/Write1/5, SPI Master Read/Write1/4, SPI Master Read/Write1/3, SPI Master Read/Write1/2
  SPI Master Read/Write1/4 -> Turn the MSB and LSB into a signed 16-bit integer GyroY/1(MSB)
  SPI Master Read/Write1/5 -> Turn the MSB and LSB into a signed 16-bit integer GyroY/2(LSB)
  SPI Master Read/Write1/6 -> Turn the MSB and LSB into a signed 16-bit integer GyroZ/1(MSB)
  SPI Master Read/Write1/7 -> Turn the MSB and LSB into a signed 16-bit integer GyroZ/2(LSB)
  SPI Master Read/Write/2 -> Turn the MSB and LSB into a signed 16-bit integer AccX/1(MSB)
  SPI Master Read/Write/3 -> Turn the MSB and LSB into a signed 16-bit integer AccX/2(LSB)
  SPI Master Read/Write/4 -> Turn the MSB and LSB into a signed 16-bit integer AccY/1(MSB)
  SPI Master Read/Write/5 -> Turn the MSB and LSB into a signed 16-bit integer AccY/2(LSB)
  SPI Master Read/Write/6 -> Turn the MSB and LSB into a signed 16-bit integer AccZ/1(MSB)
  SPI Master Read/Write/7 -> Turn the MSB and LSB into a signed 16-bit integer AccZ/2(LSB)
  Data Type Conversion1/1 -> Mux/1
  SPI Master Read/Write1/3 -> Turn the MSB and LSB into a signed 16-bit integer GyroX/1(MSB)
  SPI Master Read/Write1/2 -> Turn the MSB and LSB into a signed 16-bit integer GyroX/2(LSB)

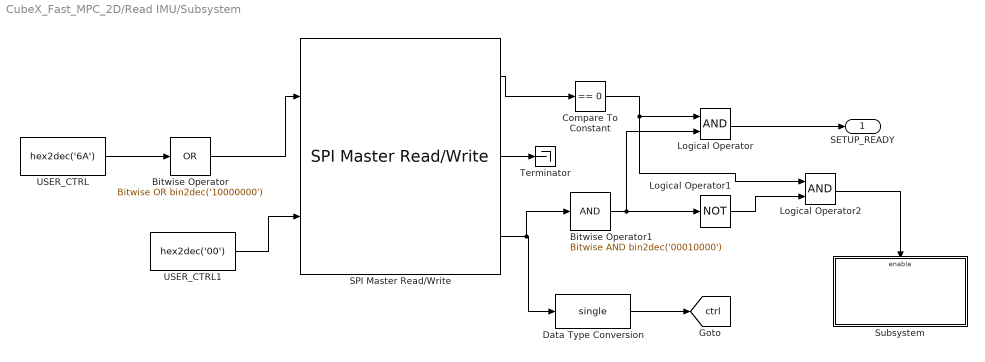
== system CubeX_Fast_MPC_2D/Read IMU/Subsystem ==
  Bitwise Operator : simulink/Logic and Bit Operations/Bitwise Operator  logicop=OR  UseBitMask=on  BitMask=bin2dec('10000000')  BitMaskRealWorld=Stored Integer
  Bitwise Operator1 : simulink/Logic and Bit Operations/Bitwise Operator  logicop=AND  UseBitMask=on  BitMask=bin2dec('00010000')  BitMaskRealWorld=Stored Integer
  Compare To Constant : simulink/Logic and Bit Operations/Compare To Constant  relop===  const=0  OutDataTypeStr=boolean
  Data Type Conversion : DataTypeConversion  OutDataTypeStr=single
  Logical Operator : Logic  AllPortsSameDT=off  OutDataTypeStr=boolean
  Logical Operator1 : Logic  Operator=NOT  AllPortsSameDT=off  OutDataTypeStr=boolean
  Logical Operator2 : Logic  AllPortsSameDT=off  OutDataTypeStr=boolean
  SPI Master Read/Write : stm32f4_spi_lib/SPI Master Read//Write  configuration=Transaction  module=3  mode=Read/ Write  lastmodule=1  direction=Full-Duplex  dataformat=8bit/ FirstBit_MSB  prescaler=4  cpolcpha=CPOL_Low/ CPHA_1Edge  datacount=2  nssmode=Custom  nsspin=Not used  softnssport=E  softnsspin=0  sckpin=A5  misopin=A6  mosipin=A7  inputtypearray=[2 3 3]  outputtypearray=[3 7 3 3]  confstr="[\"SPI_Direction_2Lines_FullDuplex\",\"8b\",\"MSB\",\"Low\",\"1Edge\",\"4\",\"Soft\",\"0\",\"x\",\"x\",\"0\",\"x\",\"x\",\"1\",\"A\",\"5\",\"1\",\"A\",\"6\",\"1\",\"A\",\"7\",\"1\",\"0\",\"0\",\"0\",\"0\",\"0\",\"0\",\"0\",\"0\",\"PP\",\"0\",\"UP\"]"  sampletime=0.002  sampletimestr=0.002  blockid=ReadIMUSubsystemSPIMasterReadWrite
  Subsystem : Subsystem
  Terminator : Terminator
  USER_CTRL : Constant  Value=hex2dec('6A')  OutDataTypeStr=uint8  SampleTime=-1
  USER_CTRL1 : Constant  Value=hex2dec('00')  OutDataTypeStr=uint8  SampleTime=-1
  SETUP_READY : Outport
  tag scope: ctrl=global
  wires:
  Bitwise Operator/1 -> SPI Master Read/Write/1
  USER_CTRL/1 -> Bitwise Operator/1
  SPI Master Read/Write/1 -> Compare To Constant/1
  Logical Operator/1 -> SETUP_READY/1
  Compare To Constant/1 -> Logical Operator/1, Logical Operator2/1
  Bitwise Operator1/1 -> Logical Operator/2, Logical Operator1/1
  Logical Operator1/1 -> Logical Operator2/2
  Logical Operator2/1 -> Subsystem/Enable
  Data Type Conversion/1 -> [ctrl]
  SPI Master Read/Write/3 -> Bitwise Operator1/1, Data Type Conversion/1
  USER_CTRL1/1 -> SPI Master Read/Write/2
  SPI Master Read/Write/2 -> Terminator/1

== system CubeX_Fast_MPC_2D/Read IMU/Accelometer Gyroscope I2C1/MPU9250 Init ==
  note: Check if BYPASS_EN bit is set in register INT_PIN_CFG
      | If not, write it in Wirte Configuration block
      |
      | With BYPASS_EN enable we can read the magnetometer data
      | from 3rd party sensor on the intern I2C bus of the MPU9250
  SlvAddr : Inport
  Bitwise Operator : simulink/Logic and Bit Operations/Bitwise Operator  logicop=AND  UseBitMask=on  BitMask=bin2dec('00000010')  BitMaskRealWorld=Stored Integer
  Compare To Zero : simulink/Logic and Bit Operations/Compare To Zero  relop===  OutDataTypeStr=boolean
  I2C Master Read/Write : stm32f4_i2c_lib/I2C Master Read//Write  configuration=Transaction  module=1  lastmodule=3  transfer=Blocking  dutycycle=TLow/THigh = 2  clkspeed=400  timeout=25  writecount=1  readcount=1  sdapin=C9  sclpin=A8  waitwritetime=0  forcestop=off  inputtypearray=[2 3 3]  outputtypearray=[2 3 3]  confstr="[\"C\",\"9\",\"A\",\"8\",\"1\",\"1\",\"6\",\"0\",\"I2C_DutyCycle_2\",\"0\",\"off\"]"  sampletime=-1  sampletimestr=0.008  blockid=ReadIMUAccelometerGyroscopeI2C1MPU9250InitI2CMasterReadWrite
  INT_PIN_CFG : Constant  Value=hex2dec('37')  OutDataTypeStr=uint8  SampleTime=-1
  Logical Operator : Logic  AllPortsSameDT=off  OutDataTypeStr=boolean
  Logical Operator1 : Logic  Operator=NOT  AllPortsSameDT=off  OutDataTypeStr=boolean
  Logical Operator2 : Logic  AllPortsSameDT=off  OutDataTypeStr=boolean
  Write Configuration : Subsystem
  SETUP_READY : Outport
  wires:
  I2C Master Read/Write/1 -> Compare To Zero/1
  INT_PIN_CFG/1 -> I2C Master Read/Write/2
  SlvAddr/1 -> Write Configuration/1(SlvAddr), I2C Master Read/Write/1
  Logical Operator/1 -> SETUP_READY/1
  Compare To Zero/1 -> Logical Operator2/1, Logical Operator/1
  Bitwise Operator/1 -> Logical Operator1/1, Logical Operator/2
  Logical Operator1/1 -> Logical Operator2/2
  Logical Operator2/1 -> Write Configuration/Enable
  I2C Master Read/Write/2 -> Bitwise Operator/1

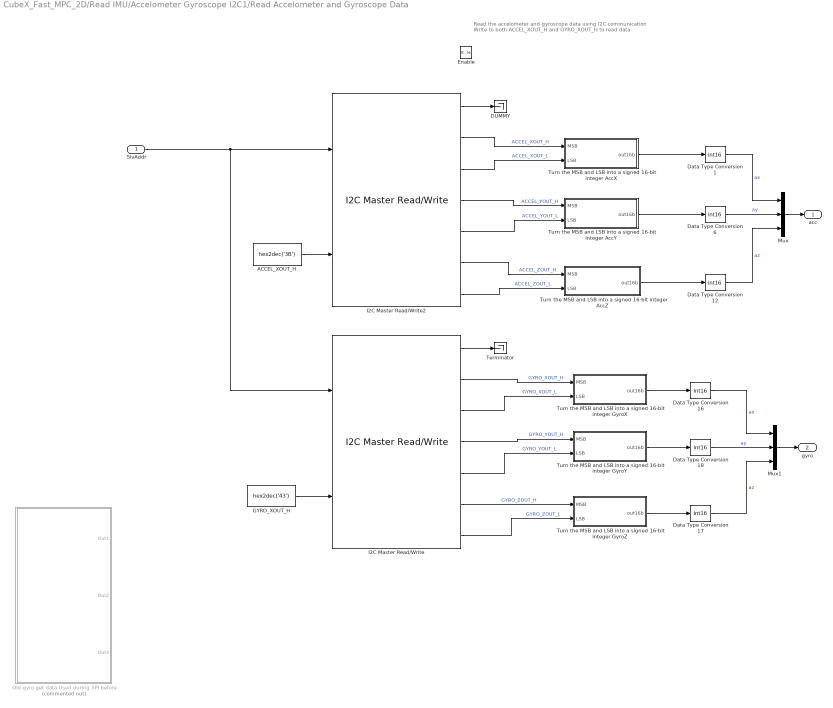
== system CubeX_Fast_MPC_2D/Read IMU/Accelometer Gyroscope I2C1/Read Accelometer and Gyroscope Data ==
  note: Read the accelometer and gyroscope data using I2C communication
      | Write to both ACCEL_XOUT_H and GYRO_XOUT_H to read data
  SlvAddr : Inport
  Enable : EnablePort
  ACCEL_XOUT_H : Constant  Value=hex2dec('3B')  OutDataTypeStr=uint8  SampleTime=-1
  DUMMY : Terminator
  Data Type Conversion{1,6,12,16..18} (6 alike) : DataTypeConversion  OutDataTypeStr=int16
  GYRO_XOUT_H : Constant  Value=hex2dec('43')  OutDataTypeStr=uint8  SampleTime=-1
  I2C Master Read/Write : stm32f4_i2c_lib/I2C Master Read//Write  configuration=Transaction  module=1  lastmodule=3  transfer=Blocking  dutycycle=TLow/THigh = 2  clkspeed=400  timeout=25  writecount=1  readcount=6  sdapin=C9  sclpin=A8  waitwritetime=0  forcestop=off  inputtypearray=[2 3 3]  outputtypearray=[7 3 3 3 3 3 3 3]  confstr="[\"C\",\"9\",\"A\",\"8\",\"1\",\"1\",\"6\",\"0\",\"I2C_DutyCycle_2\",\"0\",\"off\"]"  sampletime=Ts.IMU  sampletimestr=0.008  blockid=ReadIMUAccelometerGyroscopeI2C1ReadAccelometerandGyroscopeDataI2CMasterReadWrite
  I2C Master Read/Write2 : stm32f4_i2c_lib/I2C Master Read//Write  configuration=Transaction  module=1  lastmodule=3  transfer=Blocking  dutycycle=TLow/THigh = 2  clkspeed=400  timeout=25  writecount=1  readcount=6  sdapin=C9  sclpin=A8  waitwritetime=0  forcestop=off  inputtypearray=[2 3 3]  outputtypearray=[7 3 3 3 3 3 3 3]  confstr="[\"C\",\"9\",\"A\",\"8\",\"1\",\"1\",\"6\",\"0\",\"I2C_DutyCycle_2\",\"0\",\"off\"]"  sampletime=Ts.IMU  sampletimestr=0.008  blockid=ReadIMUAccelometerGyroscopeI2C1ReadAccelometerandGyroscopeDataI2CMasterReadWrite2
  Mux : Mux  Inputs=3
  Mux1 : Mux  Inputs=3
  Old gyro get data Used during SPI before : Subsystem  Commented=on
  Terminator : Terminator
  Turn the MSB and LSB into a signed 16-bit integer AccX : Subsystem
  Turn the MSB and LSB into a signed 16-bit integer AccY : Subsystem
  Turn the MSB and LSB into a signed 16-bit integer AccZ : Subsystem
  Turn the MSB and LSB into a signed 16-bit integer GyroX : Subsystem
  Turn the MSB and LSB into a signed 16-bit integer GyroY : Subsystem
  Turn the MSB and LSB into a signed 16-bit integer GyroZ : Subsystem
  acc : Outport
  gyro : Outport  Port=2
  wires:
  I2C Master Read/Write2/1 -> DUMMY/1
  Mux/1 -> acc/1
  Turn the MSB and LSB into a signed 16-bit integer AccX/1(out16b) -> Data Type Conversion1/1
  Turn the MSB and LSB into a signed 16-bit integer AccY/1(out16b) -> Data Type Conversion6/1
  Turn the MSB and LSB into a signed 16-bit integer AccZ/1(out16b) -> Data Type Conversion12/1
  Data Type Conversion1/1 -> Mux/1  "ax"
  Data Type Conversion6/1 -> Mux/2  "ay"
  Data Type Conversion12/1 -> Mux/3  "az"
  Mux1/1 -> gyro/1
  Turn the MSB and LSB into a signed 16-bit integer GyroX/1(out16b) -> Data Type Conversion16/1
  Turn the MSB and LSB into a signed 16-bit integer GyroY/1(out16b) -> Data Type Conversion18/1
  Turn the MSB and LSB into a signed 16-bit integer GyroZ/1(out16b) -> Data Type Conversion17/1
  Data Type Conversion16/1 -> Mux1/1  "ax"
  Data Type Conversion18/1 -> Mux1/2  "ay"
  Data Type Conversion17/1 -> Mux1/3  "az"
  GYRO_XOUT_H/1 -> I2C Master Read/Write/2
  ACCEL_XOUT_H/1 -> I2C Master Read/Write2/2
  SlvAddr/1 -> I2C Master Read/Write/1, I2C Master Read/Write2/1
  I2C Master Read/Write2/2 -> Turn the MSB and LSB into a signed 16-bit integer AccX/1(MSB)  "ACCEL_XOUT_H"
  I2C Master Read/Write2/3 -> Turn the MSB and LSB into a signed 16-bit integer AccX/2(LSB)  "ACCEL_XOUT_L"
  I2C Master Read/Write2/5 -> Turn the MSB and LSB into a signed 16-bit integer AccY/2(LSB)  "ACCEL_YOUT_L"
  I2C Master Read/Write2/4 -> Turn the MSB and LSB into a signed 16-bit integer AccY/1(MSB)  "ACCEL_YOUT_H"
  I2C Master Read/Write2/6 -> Turn the MSB and LSB into a signed 16-bit integer AccZ/1(MSB)  "ACCEL_ZOUT_H"
  I2C Master Read/Write2/7 -> Turn the MSB and LSB into a signed 16-bit integer AccZ/2(LSB)  "ACCEL_ZOUT_L"
  I2C Master Read/Write/2 -> Turn the MSB and LSB into a signed 16-bit integer GyroX/1(MSB)  "GYRO_XOUT_H"
  I2C Master Read/Write/3 -> Turn the MSB and LSB into a signed 16-bit integer GyroX/2(LSB)  "GYRO_XOUT_L"
  I2C Master Read/Write/4 -> Turn the MSB and LSB into a signed 16-bit integer GyroY/1(MSB)  "GYRO_YOUT_H"
  I2C Master Read/Write/5 -> Turn the MSB and LSB into a signed 16-bit integer GyroY/2(LSB)  "GYRO_YOUT_L"
  I2C Master Read/Write/6 -> Turn the MSB and LSB into a signed 16-bit integer GyroZ/1(MSB)  "GYRO_ZOUT_H"
  I2C Master Read/Write/7 -> Turn the MSB and LSB into a signed 16-bit integer GyroZ/2(LSB)  "GYRO_ZOUT_L"
  I2C Master Read/Write/1 -> Terminator/1

== system CubeX_Fast_MPC_2D/Read IMU/Accelometer Gyroscope I2C3/MPU9250 Init ==
  note: Check if BYPASS_EN bit is set in register INT_PIN_CFG
      | If not, write it in Wirte Configuration block
      |
      | With BYPASS_EN enable we can read the magnetometer data
      | from 3rd party sensor on the intern I2C bus of the MPU9250
  SlvAddr : Inport
  Bitwise Operator : simulink/Logic and Bit Operations/Bitwise Operator  logicop=AND  UseBitMask=on  BitMask=bin2dec('00000010')  BitMaskRealWorld=Stored Integer
  Compare To Zero : simulink/Logic and Bit Operations/Compare To Zero  relop===  OutDataTypeStr=boolean
  I2C Master Read/Write : stm32f4_i2c_lib/I2C Master Read//Write  configuration=Transaction  module=3  lastmodule=3  transfer=Blocking  dutycycle=TLow/THigh = 2  clkspeed=400  timeout=25  writecount=1  readcount=1  sdapin=C9  sclpin=A8  waitwritetime=0  forcestop=off  inputtypearray=[2 3 3]  outputtypearray=[2 3 3]  confstr="[\"C\",\"9\",\"A\",\"8\",\"1\",\"3\",\"4\",\"2\",\"I2C_DutyCycle_2\",\"0\",\"off\"]"  sampletime=-1  sampletimestr=0.008  blockid=ReadIMUAccelometerGyroscopeI2C3MPU9250InitI2CMasterReadWrite
  INT_PIN_CFG : Constant  Value=hex2dec('37')  OutDataTypeStr=uint8  SampleTime=-1
  Logical Operator : Logic  AllPortsSameDT=off  OutDataTypeStr=boolean
  Logical Operator1 : Logic  Operator=NOT  AllPortsSameDT=off  OutDataTypeStr=boolean
  Logical Operator2 : Logic  AllPortsSameDT=off  OutDataTypeStr=boolean
  Write Configuration : Subsystem
  SETUP_READY : Outport
  wires:
  I2C Master Read/Write/1 -> Compare To Zero/1
  INT_PIN_CFG/1 -> I2C Master Read/Write/2
  SlvAddr/1 -> Write Configuration/1(SlvAddr), I2C Master Read/Write/1
  Logical Operator/1 -> SETUP_READY/1
  Compare To Zero/1 -> Logical Operator2/1, Logical Operator/1
  Bitwise Operator/1 -> Logical Operator1/1, Logical Operator/2
  Logical Operator1/1 -> Logical Operator2/2
  Logical Operator2/1 -> Write Configuration/Enable
  I2C Master Read/Write/2 -> Bitwise Operator/1
